simulink model "test_fastterminal_formation_gazebo_paper_cts23a"  (R2023a)
settings: Solver=FixedStepAuto  StartTime=0.0  StopTime=inf  RelTol=1e-3
undefined symbols (not defined in the file or in its folder): angular, DiscIntNeverNeededParam, linear
libraries: ros2lib x11, simulink x4, robotcorelib x4
(part 2 of 2)

== matlab function test_fastterminal_formation_gazebo_paper_cts23a/Translational Control3/Flocking1/MATLAB Function2 ==
  data: xi input; yi input; zi input; dxi input; dyi input; dzi input; U output; xr input; yr input; zr input; dxr input; dyr input; dzr input; xr2 input; yr2 input; zr2 input; dxr2 input; dyr2 input; dzr2 input; xr3 input; yr3 input; zr3 input; dxr3 input; dyr3 input; dzr3 input; iep input size=3; ep output size=3; S output; E output; K_cts input; S_cts input; NN input

function [U, ep, S, E] = naviFeedback(xi, yi, zi, dxi, dyi, dzi, xr, yr, zr, dxr, dyr, dzr, xr2, yr2, zr2, dxr2, dyr2, dzr2, xr3, yr3, zr3, dxr3, dyr3, dzr3, iep, K_cts, S_cts, NN)
    
    Kp = K_cts(1); Kpz = K_cts(2);

    % Cts manifold
    C1_xy = S_cts(1); C2_xy = S_cts(2); alpha1_xy = S_cts(3); alpha2_xy = S_cts(4);
    C1_z = S_cts(5); C2_z = S_cts(6); alpha1_z = S_cts(7); alpha2_z = S_cts(8);
    
    %errors
    ex = (xr2 - xi) + (xr3 - xi - 0.25);
    ey = (yr2 - yi + 0.86) + (yr3 - yi + 0.43);
    ez = (zr2 - zi) + (zr3 - zi);
    ep = [ex;ey;ez];

    dex = (dxr2 - dxi) + (dxr3 - dxi);
    dey = (dyr2 - dyi) + (dyr3 - dxi);
    dez = (dzr2 - dzi) + (dzr3 - dxi);
    E = [ex;ey;ez;dex;dey;dez];

    %error integrals
    iex = iep(1);
    iey = iep(2);
    iez = iep(3);
    
    %Manifold definitions
    Sx = manifold_pos_int(iex, ex, C1_xy, C2_xy, alpha1_xy, alpha2_xy);
    Sy = manifold_pos_int(iey, ey, C1_xy, C2_xy, alpha1_xy, alpha2_xy);
    Sz = manifold_pos_int(iez, ez, C1_z, C2_z, alpha1_z, alpha2_z);

    S = [Sx;Sy;Sz];

    ux = fast_con2(iex, ex, Sx, dxr + dxr2 + dxr3, C1_xy, C2_xy, alpha1_xy, alpha2_xy, Kp) - NN(1);
    uy = fast_con2(iey, ey, Sy, dyr + dyr2 + dyr3, C1_xy, C2_xy, alpha1_xy, alpha2_xy, Kp) - NN(2);
    uz = fast_con2(iez, ez, Sz, dzr + dzr2 + dzr3, C1_z, C2_z, alpha1_z, alpha2_z, Kpz) - NN(3);

    U = [ux;uy;uz];
end

== matlab function test_fastterminal_formation_gazebo_paper_cts23a/Extract pose 1/Observer_for_speed ==
  data: X input; dXhat_1 output; Xhat input; Xhat2 input; K1ob input; K2ob input; dXhat_2 output
function [dXhat_1, dXhat_2] = fcn(X, Xhat, Xhat2, K1ob, K2ob)

%%
%Separation of the actual states
X_a = X(1:3);
x = X_a(1);  y = X_a(2);  z = X_a(3);    

%%
%Estimation vector separation
X_hat = Xhat(1:3);
x_h1 = X_hat(1);
y_h1 = X_hat(2);
z_h1 = X_hat(3);

%%
%Observer errors definition
e_x = x - x_h1;
e_y = y - y_h1;
e_z = z - z_h1;

%%
%Vector form
e_X = [e_x;e_y;e_z];

pow = [0.5;0.5;0.5];

%%
%Computation of the observer
dXhat_1 = Xhat2 + (K1ob*abs(e_X).^pow).*tanh(e_X);
dXhat_2 = K2ob*tanh(e_X);

== matlab function test_fastterminal_formation_gazebo_paper_cts23a/Translational Control2/Flocking1/OFC1 ==
  settings: updateMethod=DISCRETE  sampleTime=0.05
  data: OFC output size=1; dW output; s input; E input; W input; bel input
function [OFC,dW] = fcn(s, E,W, bel)

m = 70;
sigma = bel(1); %12
alpha_ofc = bel(2); %1
r1 = bel(3);
r2 = bel(4);

%Sliding
sx = s(1,1);

ex = E(1,1);
dex = E(4,1);

persistent phivec

if isempty(phivec)
    phivec = zeros(m,1);
end

mu1 = linspace(-r1, r1, m); 
mu2 = linspace(-r2, r2, m); 

for i = 1:1:m
    phivec(i) = exp(-(norm(ex-mu1(i))^2+norm(dex-mu2(i))^2)/(sigma^2));
end

OFC = W'*phivec;

dW = -alpha_ofc*sx*phivec;

== matlab function test_fastterminal_formation_gazebo_paper_cts23a/Translational Control2/Flocking1/OFC2 ==
  settings: updateMethod=DISCRETE  sampleTime=0.05
  data: OFC output size=1; dW output; s input; E input; W input; bel input
function [OFC,dW] = fcn(s, E,W, bel)

m = 70;
sigma = bel(1); %12
alpha_ofc = bel(2); %1
r1 = bel(3);
r2 = bel(4);

%Sliding
sy = s(2,1);

ey = E(2,1);
dey = E(5,1);

persistent phivec

if isempty(phivec)
    phivec = zeros(m,1);
end

mu1 = linspace(-r1, r1, m);
mu2 = linspace(-r2, r2, m);

for i = 1:1:m
    phivec(i) = exp(-(norm(ey-mu1(i))^2+norm(dey-mu2(i))^2)/(sigma^2));
end

OFC = W'*phivec;

dW = -alpha_ofc*sy*phivec;

== matlab function test_fastterminal_formation_gazebo_paper_cts23a/Translational Control2/Flocking1/OFC3 ==
  settings: updateMethod=DISCRETE  sampleTime=0.05
  data: OFC output size=1; dW output; s input; E input; W input; bel input
function [OFC,dW] = fcn(s, E, W, bel)

m = 70;
sigma = bel(5); %12
alpha_ofc = bel(6); %1
r1 = bel(7);
r2 = bel(8);

%Sliding
sz = s(3,1);

ez = E(3,1);
dez = E(6,1);

persistent phivec

if isempty(phivec)
    phivec = zeros(m,1);
end

mu1 = linspace(-r1, r1, m); 
mu2 = linspace(-r2, r2, m); 

for i = 1:1:m
    phivec(i) = exp(-(norm(ez-mu1(i))^2+norm(dez-mu2(i))^2)/(sigma^2));
end

OFC = W'*phivec;

dW = -alpha_ofc*sz*phivec;

== matlab function test_fastterminal_formation_gazebo_paper_cts23a/Translational Control1/Flocking1/MATLAB Function ==
  data: xi input; yi input; phiAlpha output; xj input; yj input; xk input; yk input; xl input; yl input; params input

function phiAlpha  = phiAlphaFcn(xi, yi, xj, yj, xk, yk, xl, yl, params)
    
    % Flocking parameters
    epsilon = params(1); a = params(2); b = params(3); c = params(4); d = params(5); h = params(6);

    e = abs(a - b) / sqrt(4*a*b) ;

    cAlpha = sigmaNormFun(c, epsilon) ;
    dAlpha = sigmaNormFun(d, epsilon) ;

    %%
    Pi = [xi;yi] ;
    Pj = [xj;yj] ;
    Pk = [xk;yk] ;
    Pl = [xl;yl] ;

    %%
    sigmaNormj = sigmaNormFun(Pj - Pi, epsilon) ;
    nij = gradSigmaFun(Pj - Pi, epsilon) ;
    
    sigmaNormk = sigmaNormFun(Pk - Pi, epsilon) ;
    nik = gradSigmaFun(Pk - Pi, epsilon) ;

    sigmaNorml = sigmaNormFun(Pl - Pi, epsilon) ;
    nil = gradSigmaFun(Pl - Pi, epsilon) ;

    %%
    sigma1j = sigma1Fun(sigmaNormj - dAlpha + e) ;
    sigma1k = sigma1Fun(sigmaNormk - dAlpha + e) ;
    sigma1l = sigma1Fun(sigmaNorml - dAlpha + e) ;
            
    %% Position
    phiAlphaj = 0.5 * bumpFcn(sigmaNormj/cAlpha,h) * ((a+b)*sigma1j + (a-b)) ;
    phiAlphanij = phiAlphaj.* nij ;
    
    phiAlphak = 0.5 * bumpFcn(sigmaNormk/cAlpha,h) * ((a+b)*sigma1k + (a-b)) ;
    phiAlphanik = phiAlphak.* nik ;

    phiAlphal = 0.5 * bumpFcn(sigmaNorml/cAlpha,h) * ((a+b)*sigma1l + (a-b)) ;
    phiAlphanil = phiAlphal.* nil ;

    phiAlpha = phiAlphanij + phiAlphanik + phiAlphanil;

    
end

== matlab function test_fastterminal_formation_gazebo_paper_cts23a/Translational Control1/Flocking1/MATLAB Function1 ==
  data: phiAlpha input; phiAlpha_int input; ui_gamma input; yaw input; KP input; syaw input; Ui_pos output size=3; ui_yaw output; eyaw output; eyaw2 input; eyaw3 input

function [Ui_pos, ui_yaw, eyaw]  = ctrlLaw(phiAlpha, phiAlpha_int, ui_gamma, yaw, KP, syaw, eyaw2, eyaw3)  
    
    % Control gains and parameters
    k1 = syaw(1); sigma = syaw(2); beta = syaw(3); 
    ks = syaw(4); ke = syaw(5);

    % Control gains and parameters
    Kx = KP(1); Ky = KP(2); Kz = KP(3);
    Kix = KP(4); Kiy = KP(5); Kiz = KP(6);
    Kyaw = KP(7); Kdyaw = KP(8); Kiyaw = KP(9);
    offset = KP(10);
    
    eyaw = 0 - yaw(1);
    deyaw = 0 - yaw(2);

    %Manifold
    Syaw = manifold_ter_back_yaw(eyaw, deyaw, sigma, beta);
    %Control
    ui_yaw = back_ter_yaw_con(eyaw, Syaw, sigma, beta, k1, ks, ke);
    hz_dot = ui_gamma(3,1);  %

    if eyaw < offset && eyaw > -offset && eyaw2 < offset && eyaw2 > -offset && eyaw3 < offset && eyaw3 > -offset 
        hx_dot =  ui_gamma(1,1);  %Kx * phiAlpha(1,1) + Kix * phiAlpha_int(1,1) + 
        hy_dot =  ui_gamma(2,1);  %Ky * phiAlpha(2,1) + Kiy * phiAlpha_int(2,1) + 
    else
        hx_dot =  0;  %
        hy_dot =  0;  %
    end    

    Ui_pos = [hx_dot; hy_dot; hz_dot] ;
    

end

== matlab function test_fastterminal_formation_gazebo_paper_cts23a/Translational Control1/Flocking1/MATLAB Function2 ==
  data: xi input; yi input; zi input; dxi input; dyi input; dzi input; U output; xr input; yr input; zr input; dxr input; dyr input; dzr input; iep input size=3; ep output size=3; S output; E output; K_cts input; S_cts input; NN input

function [U, ep, S, E] = naviFeedback(xi, yi, zi, dxi, dyi, dzi, xr, yr, zr, dxr, dyr, dzr, iep, K_cts, S_cts, NN)
    
    Kp = K_cts(1); Kpz = K_cts(2);

    % Cts manifold
    C1_xy = S_cts(1); C2_xy = S_cts(2); alpha1_xy = S_cts(3); alpha2_xy = S_cts(4);
    C1_z = S_cts(5); C2_z = S_cts(6); alpha1_z = S_cts(7); alpha2_z = S_cts(8);
    
    %errors
    ex = (xr - xi + 0.5);
    ey = (yr - yi);
    ez = (zr - zi);
    ep = [ex;ey;ez];

    dex = (dxr - dxi);
    dey = (dyr - dyi);
    dez = (dzr - dzi);
    E = [ex;ey;ez;dex;dey;dez];

    %error integrals
    iex = iep(1);
    iey = iep(2);
    iez = iep(3);
    
    %Manifold definitions
    Sx = manifold_pos_int(iex, ex, C1_xy, C2_xy, alpha1_xy, alpha2_xy);
    Sy = manifold_pos_int(iey, ey, C1_xy, C2_xy, alpha1_xy, alpha2_xy);
    Sz = manifold_pos_int(iez, ez, C1_z, C2_z, alpha1_z, alpha2_z);

    S = [Sx;Sy;Sz];

    ux = fast_con2(iex, ex, Sx, dxr, C1_xy, C2_xy, alpha1_xy, alpha2_xy, Kp) - NN(1);
    uy = fast_con2(iey, ey, Sy, dyr, C1_xy, C2_xy, alpha1_xy, alpha2_xy, Kp) - NN(2);
    uz = fast_con2(iez, ez, Sz, dzr, C1_z, C2_z, alpha1_z, alpha2_z, Kpz) - NN(3);

    U = [ux;uy;uz];
end

== matlab function test_fastterminal_formation_gazebo_paper_cts23a/Extract pose 2/Observer_for_speed ==
  data: X input; dXhat_1 output; Xhat input; Xhat2 input; K1ob input; K2ob input; dXhat_2 output
function [dXhat_1, dXhat_2] = fcn(X, Xhat, Xhat2, K1ob, K2ob)

%%
%Separation of the actual states
X_a = X(1:3);
x = X_a(1);  y = X_a(2);  z = X_a(3);    

%%
%Estimation vector separation
X_hat = Xhat(1:3);
x_h1 = X_hat(1);
y_h1 = X_hat(2);
z_h1 = X_hat(3);

%%
%Observer errors definition
e_x = x - x_h1;
e_y = y - y_h1;
e_z = z - z_h1;

%%
%Vector form
e_X = [e_x;e_y;e_z];

pow = [0.5;0.5;0.5];

%%
%Computation of the observer
dXhat_1 = Xhat2 + (K1ob*abs(e_X).^pow).*tanh(e_X);
dXhat_2 = K2ob*tanh(e_X);

== matlab function test_fastterminal_formation_gazebo_paper_cts23a/Extract pose 3/Observer_for_speed ==
  data: X input; dXhat_1 output; Xhat input; Xhat2 input; K1ob input; K2ob input; dXhat_2 output
function [dXhat_1, dXhat_2] = fcn(X, Xhat, Xhat2, K1ob, K2ob)

%%
%Separation of the actual states
X_a = X(1:3);
x = X_a(1);  y = X_a(2);  z = X_a(3);    

%%
%Estimation vector separation
X_hat = Xhat(1:3);
x_h1 = X_hat(1);
y_h1 = X_hat(2);
z_h1 = X_hat(3);

%%
%Observer errors definition
e_x = x - x_h1;
e_y = y - y_h1;
e_z = z - z_h1;

%%
%Vector form
e_X = [e_x;e_y;e_z];

pow = [0.5;0.5;0.5];

%%
%Computation of the observer
dXhat_1 = Xhat2 + (K1ob*abs(e_X).^pow).*tanh(e_X);
dXhat_2 = K2ob*tanh(e_X);

== matlab function test_fastterminal_formation_gazebo_paper_cts23a/Translational Control3/Flocking1/OFC1 ==
  settings: updateMethod=DISCRETE  sampleTime=0.05
  data: OFC output size=1; dW output; s input; E input; W input; bel input
function [OFC,dW] = fcn(s, E,W, bel)

m = 70;
sigma = bel(1); %12
alpha_ofc = bel(2); %1
r1 = bel(3);
r2 = bel(4);

%Sliding
sx = s(1,1);

ex = E(1,1);
dex = E(4,1);

persistent phivec

if isempty(phivec)
    phivec = zeros(m,1);
end

mu1 = linspace(-r1, r1, m); 
mu2 = linspace(-r2, r2, m); 

for i = 1:1:m
    phivec(i) = exp(-(norm(ex-mu1(i))^2+norm(dex-mu2(i))^2)/(sigma^2));
end

OFC = W'*phivec;

dW = -alpha_ofc*sx*phivec;

== matlab function test_fastterminal_formation_gazebo_paper_cts23a/Translational Control3/Flocking1/OFC2 ==
  settings: updateMethod=DISCRETE  sampleTime=0.05
  data: OFC output size=1; dW output; s input; E input; W input; bel input
function [OFC,dW] = fcn(s, E,W, bel)

m = 70;
sigma = bel(1); %12
alpha_ofc = bel(2); %1
r1 = bel(3);
r2 = bel(4);

%Sliding
sy = s(2,1);

ey = E(2,1);
dey = E(5,1);

persistent phivec

if isempty(phivec)
    phivec = zeros(m,1);
end

mu1 = linspace(-r1, r1, m);
mu2 = linspace(-r2, r2, m);

for i = 1:1:m
    phivec(i) = exp(-(norm(ey-mu1(i))^2+norm(dey-mu2(i))^2)/(sigma^2));
end

OFC = W'*phivec;

dW = -alpha_ofc*sy*phivec;

== matlab function test_fastterminal_formation_gazebo_paper_cts23a/Translational Control3/Flocking1/OFC3 ==
  settings: updateMethod=DISCRETE  sampleTime=0.05
  data: OFC output size=1; dW output; s input; E input; W input; bel input
function [OFC,dW] = fcn(s, E, W, bel)

m = 70;
sigma = bel(5); %12
alpha_ofc = bel(6); %1
r1 = bel(7);
r2 = bel(8);

%Sliding
sz = s(3,1);

ez = E(3,1);
dez = E(6,1);

persistent phivec

if isempty(phivec)
    phivec = zeros(m,1);
end

mu1 = linspace(-r1, r1, m); 
mu2 = linspace(-r2, r2, m); 

for i = 1:1:m
    phivec(i) = exp(-(norm(ez-mu1(i))^2+norm(dez-mu2(i))^2)/(sigma^2));
end

OFC = W'*phivec;

dW = -alpha_ofc*sz*phivec;

== matlab function test_fastterminal_formation_gazebo_paper_cts23a/continuous ==
  data: i output; t input; tp input; tp output; i input
function [i,tp] = fcn(t,tp,i)


%u = 0.1*cos(1.5*t) + 0.05*sin(t);         % x-component of vector field
%v = 0.1*sin(3*t) - 0.06*sin(0.5*t);      % y-component of vector field
if t > tp
    i = i + 1;
else 
    i = i;
end

== matlab function test_fastterminal_formation_gazebo_paper_cts23a/MATLAB Function1 ==
  data: sec input; gaz_time output; nanosec input
function gaz_time = fcn(sec, nanosec)

nanosec1 = double(nanosec)/1000000000; %*10^(-9);

sec1 = double(sec);

gaz_time = sec1 + nanosec1;
